simulink model "task3"  (R2023a)
settings: Solver=VariableStepAuto  StartTime=0.0  StopTime=10.0  RelTol=1e-3
settings Model: Creator=17634948724  LastModifiedBy=17634948724

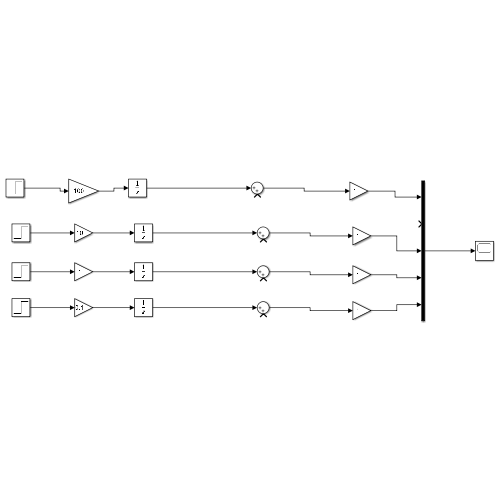
[thumbnail: Simulink's stored preview of the top-level diagram]
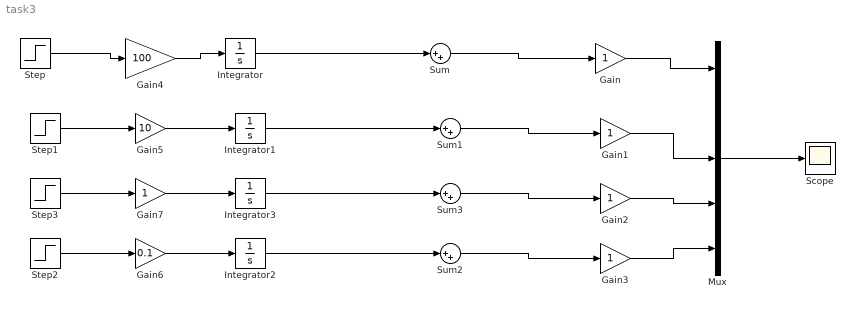
== system task3 ==
  Gain{,1..3,7} (5 alike) : Gain
  Gain4 : Gain  Gain=100
  Gain5 : Gain  Gain=10
  Gain6 : Gain  Gain=0.1
  Integrator{,1..3} (4 alike) : Integrator
  Mux : Mux  Inputs=5
  Scope : Scope
  Step{,1..3} (4 alike) : Step  Time=0  SampleTime=0
  Sum{,1..3} (4 alike) : Sum  Inputs=|++
  wires:
  Step/1 -> Gain4/1
  Integrator/1 -> Sum/1
  Sum/1 -> Gain/1
  Gain2/1 -> Mux/4
  Mux/1 -> Scope/1
  Gain4/1 -> Integrator/1
  Step1/1 -> Gain5/1
  Integrator1/1 -> Sum1/1
  Gain5/1 -> Integrator1/1
  Sum1/1 -> Gain1/1
  Step3/1 -> Gain7/1
  Integrator3/1 -> Sum3/1
  Gain7/1 -> Integrator3/1
  Sum3/1 -> Gain2/1
  Sum2/1 -> Gain3/1
  Gain6/1 -> Integrator2/1
  Integrator2/1 -> Sum2/1
  Step2/1 -> Gain6/1
  Gain3/1 -> Mux/5
  Gain1/1 -> Mux/3
  Gain/1 -> Mux/1
